simulink model "Point_3"  (R2024b)
settings: Solver=ode45  StartTime=0.0  StopTime=Tf  FixedStep=0.01  RelTol=1e-7
libraries: robotmobilelib x2
settings Model: Creator=emanuela  LastModifiedBy=emanuela

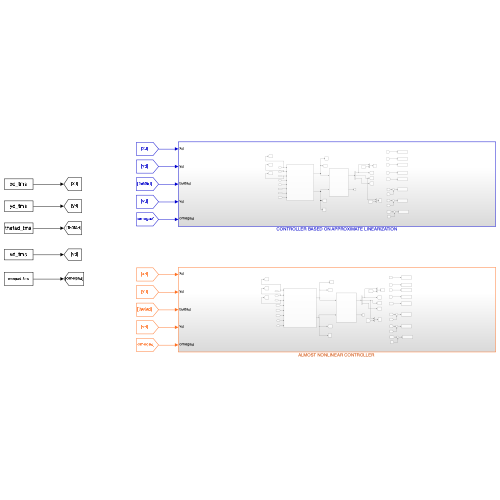
[thumbnail: Simulink's stored preview of the top-level diagram]
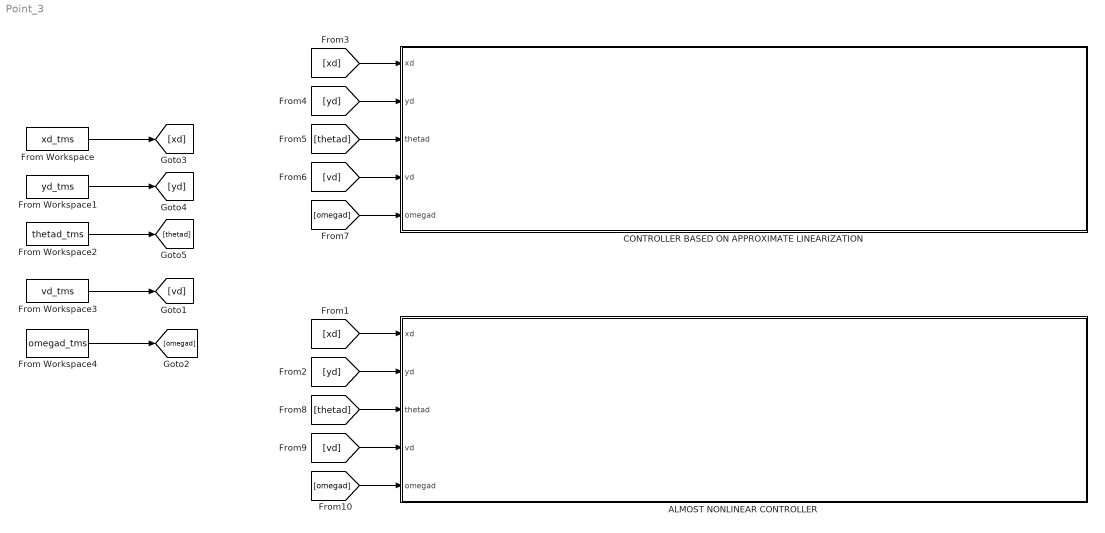
== system Point_3 ==
  "ALMOST NONLINEAR CONTROLLER " : Subsystem
  CONTROLLER BASED ON APPROXIMATE LINEARIZATION : Subsystem
  From Workspace : FromWorkspace  VariableName=xd_tms
  From Workspace1 : FromWorkspace  VariableName=yd_tms
  From Workspace2 : FromWorkspace  VariableName=thetad_tms
  From Workspace3 : FromWorkspace  VariableName=vd_tms
  From Workspace4 : FromWorkspace  VariableName=omegad_tms
  wires:
  From Workspace/1 -> [xd]
  From Workspace1/1 -> [yd]
  From Workspace2/1 -> [thetad]
  From Workspace3/1 -> [vd]
  From Workspace4/1 -> [omegad]
  [xd] -> CONTROLLER BASED ON APPROXIMATE LINEARIZATION/1(xd)
  [yd] -> CONTROLLER BASED ON APPROXIMATE LINEARIZATION/2(yd)
  [thetad] -> CONTROLLER BASED ON APPROXIMATE LINEARIZATION/3(thetad)
  [vd] -> CONTROLLER BASED ON APPROXIMATE LINEARIZATION/4(vd)
  [omegad] -> CONTROLLER BASED ON APPROXIMATE LINEARIZATION/5(omegad)
  [yd] -> "ALMOST NONLINEAR CONTROLLER "/2(yd)
  [omegad] -> "ALMOST NONLINEAR CONTROLLER "/5(omegad)
  [vd] -> "ALMOST NONLINEAR CONTROLLER "/4(vd)
  [xd] -> "ALMOST NONLINEAR CONTROLLER "/1(xd)
  [thetad] -> "ALMOST NONLINEAR CONTROLLER "/3(thetad)

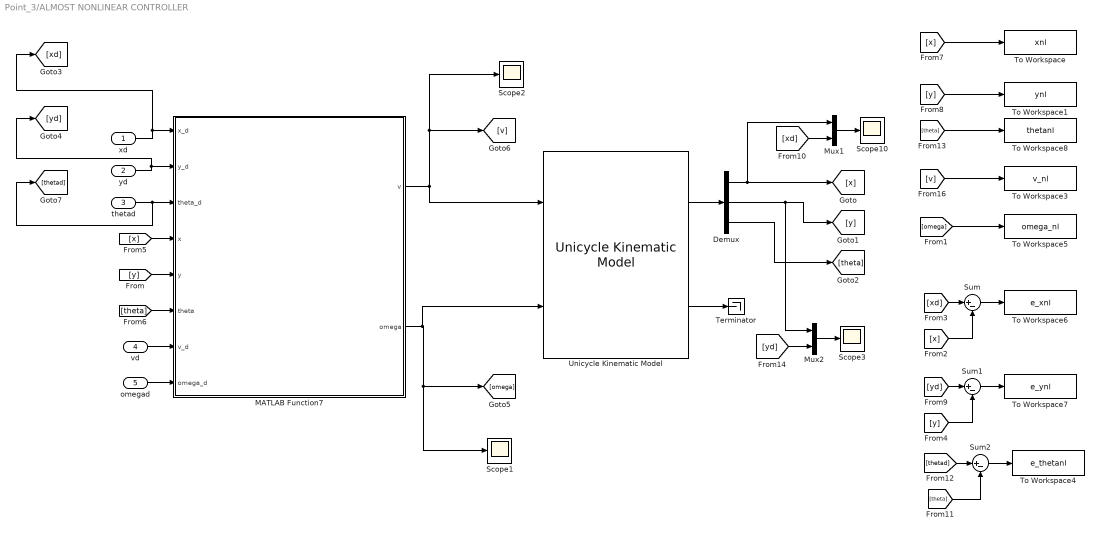
== system Point_3/ALMOST NONLINEAR CONTROLLER  ==
  xd : Inport
  yd : Inport  Port=2
  thetad : Inport  Port=3
  vd : Inport  Port=4
  omegad : Inport  Port=5
  Demux : Demux  Outputs=3
  MATLAB Function7 : MATLAB Function  TreatAsAtomicUnit=on
  Mux1 : Mux  Inputs=2
  Mux2 : Mux  Inputs=2
  Scope{1..3,10} (4 alike) : Scope
  Sum : Sum  Inputs=|+-
  Sum1 : Sum  Inputs=|+-
  Sum2 : Sum  Inputs=|+-
  Terminator : Terminator
  To Workspace : ToWorkspace  VariableName=xnl  SaveFormat=Structure With Time  SampleTime=-1
  To Workspace1 : ToWorkspace  VariableName=ynl  SaveFormat=Structure With Time  SampleTime=-1
  To Workspace3 : ToWorkspace  VariableName=v_nl  SaveFormat=Structure With Time  SampleTime=-1
  To Workspace4 : ToWorkspace  VariableName=e_thetanl  SaveFormat=Structure With Time  SampleTime=-1
  To Workspace5 : ToWorkspace  VariableName=omega_nl  SaveFormat=Structure With Time  SampleTime=-1
  To Workspace6 : ToWorkspace  VariableName=e_xnl  SaveFormat=Structure With Time  SampleTime=-1
  To Workspace7 : ToWorkspace  VariableName=e_ynl  SaveFormat=Structure With Time  SampleTime=-1
  To Workspace8 : ToWorkspace  VariableName=thetanl  SaveFormat=Structure With Time  SampleTime=-1
  Unicycle Kinematic Model : robotmobilelib/Unicycle Kinematic Model  VehicleInputs=Vehicle Speed & Heading Angular Velocity  WheelRadius=0.1  WheelSpeedRange=[-Inf Inf]  InitialState=initial_state  SimulateUsing=Interpreted execution
  wires:
  Unicycle Kinematic Model/2 -> Terminator/1
  Demux/2 -> Mux2/1, [y]
  Demux/3 -> [theta]
  Demux/1 -> Mux1/1, [x]
  xd/1 -> MATLAB Function7/1(x_d), [xd]
  yd/1 -> MATLAB Function7/2(y_d), [yd]
  MATLAB Function7/1(v) -> Scope2/1, [v], Unicycle Kinematic Model/1
  Unicycle Kinematic Model/1 -> Demux/1
  [y] -> To Workspace1/1
  [x] -> To Workspace/1
  [v] -> To Workspace3/1
  [omega] -> To Workspace5/1
  [x] -> Sum/2
  thetad/1 -> [thetad], MATLAB Function7/3(theta_d)
  [xd] -> Sum/1
  Sum/1 -> To Workspace6/1
  [yd] -> Sum1/1
  Sum1/1 -> To Workspace7/1
  [y] -> Sum1/2
  MATLAB Function7/2(omega) -> Unicycle Kinematic Model/2, Scope1/1, [omega]
  [theta] -> Sum2/2
  [theta] -> To Workspace8/1
  [thetad] -> Sum2/1
  Sum2/1 -> To Workspace4/1
  Mux1/1 -> Scope10/1
  [xd] -> Mux1/2
  [yd] -> Mux2/2
  Mux2/1 -> Scope3/1
  [x] -> MATLAB Function7/4(x)
  [y] -> MATLAB Function7/5(y)
  [theta] -> MATLAB Function7/6(theta)
  vd/1 -> MATLAB Function7/7(v_d)
  omegad/1 -> MATLAB Function7/8(omega_d)

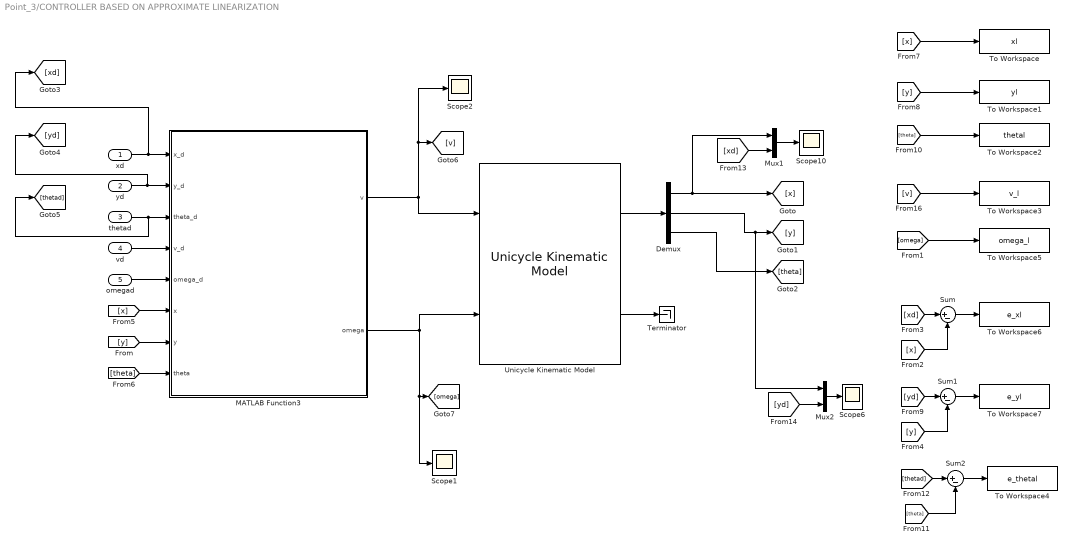
== system Point_3/CONTROLLER BASED ON APPROXIMATE LINEARIZATION ==
  xd : Inport
  yd : Inport  Port=2
  thetad : Inport  Port=3
  vd : Inport  Port=4
  omegad : Inport  Port=5
  Demux : Demux  Outputs=3
  MATLAB Function3 : MATLAB Function  TreatAsAtomicUnit=on
  Mux1 : Mux  Inputs=2
  Mux2 : Mux  Inputs=2
  Scope{1..2,6,10} (4 alike) : Scope
  Sum : Sum  Inputs=|+-
  Sum1 : Sum  Inputs=|+-
  Sum2 : Sum  Inputs=|+-
  Terminator : Terminator
  To Workspace : ToWorkspace  VariableName=xl  SaveFormat=Structure With Time  SampleTime=-1
  To Workspace1 : ToWorkspace  VariableName=yl  SaveFormat=Structure With Time  SampleTime=-1
  To Workspace2 : ToWorkspace  VariableName=thetal  SaveFormat=Structure With Time  SampleTime=-1
  To Workspace3 : ToWorkspace  VariableName=v_l  SaveFormat=Structure With Time  SampleTime=-1
  To Workspace4 : ToWorkspace  VariableName=e_thetal  SaveFormat=Structure With Time  SampleTime=-1
  To Workspace5 : ToWorkspace  VariableName=omega_l  SaveFormat=Structure With Time  SampleTime=-1
  To Workspace6 : ToWorkspace  VariableName=e_xl  SaveFormat=Structure With Time  SampleTime=-1
  To Workspace7 : ToWorkspace  VariableName=e_yl  SaveFormat=Structure With Time  SampleTime=-1
  Unicycle Kinematic Model : robotmobilelib/Unicycle Kinematic Model  VehicleInputs=Vehicle Speed & Heading Angular Velocity  WheelRadius=0.1  WheelSpeedRange=[-Inf Inf]  InitialState=initial_state  SimulateUsing=Interpreted execution
  wires:
  Unicycle Kinematic Model/2 -> Terminator/1
  Demux/2 -> Mux2/1, [y]
  Demux/3 -> [theta]
  Demux/1 -> Mux1/1, [x]
  xd/1 -> [xd], MATLAB Function3/1(x_d)
  yd/1 -> [yd], MATLAB Function3/2(y_d)
  vd/1 -> MATLAB Function3/4(v_d)
  omegad/1 -> MATLAB Function3/5(omega_d)
  [x] -> MATLAB Function3/6(x)
  [y] -> MATLAB Function3/7(y)
  [theta] -> MATLAB Function3/8(theta)
  MATLAB Function3/2(omega) -> Scope1/1, [omega], Unicycle Kinematic Model/2
  MATLAB Function3/1(v) -> Scope2/1, [v], Unicycle Kinematic Model/1
  Unicycle Kinematic Model/1 -> Demux/1
  [y] -> To Workspace1/1
  [x] -> To Workspace/1
  [v] -> To Workspace3/1
  [omega] -> To Workspace5/1
  [x] -> Sum/2
  thetad/1 -> [thetad], MATLAB Function3/3(theta_d)
  [xd] -> Sum/1
  Sum/1 -> To Workspace6/1
  [yd] -> Sum1/1
  Sum1/1 -> To Workspace7/1
  [y] -> Sum1/2
  [theta] -> To Workspace2/1
  [thetad] -> Sum2/1
  [theta] -> Sum2/2
  Sum2/1 -> To Workspace4/1
  [xd] -> Mux1/2
  Mux1/1 -> Scope10/1
  Mux2/1 -> Scope6/1
  [yd] -> Mux2/2

== matlab function Point_3/CONTROLLER BASED ON APPROXIMATE LINEARIZATION/MATLAB Function3 ==
  data: v output; x_d input; y_d input; theta_d input; v_d input; omega_d input; x input; y input; theta input; omega output
function [v,omega] = control_inputs_app_lin(x_d,y_d,theta_d,v_d,omega_d,x,y,theta)


 zita = 0.6;
 a = 1;
 k1 = 2*zita*a;
 k3 = k1;
 k2 = (a^2-0.01*abs(omega_d^2))/abs(v_d);

 M = [cos(theta) sin(theta) 0; -sin(theta) cos(theta) 0; 0 0 1];
 displacement = [x_d-x; y_d-y; theta_d-theta];
 e = M*displacement;

 u1 = -k1*e(1);
 u2 = -k2*e(2)-k3*e(3);

 v = v_d*cos(e(3))-u1;
 omega = omega_d-u2;

end

== matlab function Point_3/ALMOST NONLINEAR CONTROLLER /MATLAB Function7 ==
  data: v output; x_d input; y_d input; theta_d input; x input; y input; theta input; v_d input; omega_d input; omega output
function [v,omega] = control_inputs_almost_nl(x_d,y_d,theta_d,x,y,theta,v_d,omega_d)

%For r1=2
k1 = 3+0.2*abs(v_d)+0.1*abs(omega_d);
k2 = 3.5;  
k3 = 5+0.2*abs(omega_d)+0.3*abs(v_d);

% %For r2=0.2
% k1 = 3+0.01*abs(v_d)+0.01*abs(omega_d);
% k2 = 3.5;  
% k3 = 5+0.01*abs(omega_d)+0.01*abs(v_d);

M = [cos(theta) sin(theta) 0; -sin(theta) cos(theta) 0; 0 0 1];
displacement = [x_d-x; y_d-y; theta_d-theta];
e = M*displacement;

sinc_e3 = sin(e(3))/e(3);
u1 = -k1*e(1);
u2 = -k2*v_d*(sinc_e3)*e(2)-k3*e(3);

v = v_d*cos(e(3))-u1;
omega = omega_d-u2;

end
